simulink model "test_increase_button_laterelease"  (R2022b)
settings: Solver=FixedStepAuto  StartTime=0.0  StopTime=240  FixedStep=0.1  RelTol=1e-3
settings Model: Creator=cristian  LastModifiedBy=cristian
settings ConfigComp: CovEnable=on  RecordCoverage=on  CovModelRefEnable=on

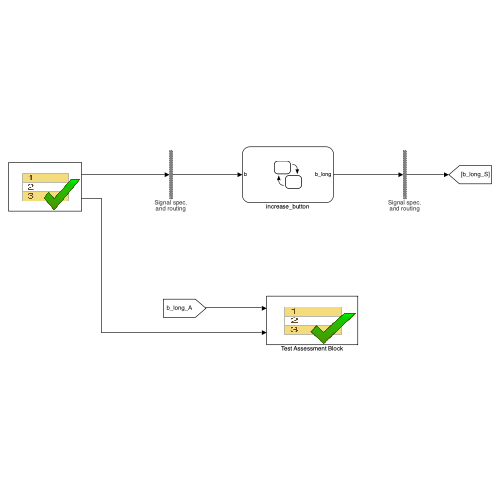
[thumbnail: Simulink's stored preview of the top-level diagram]
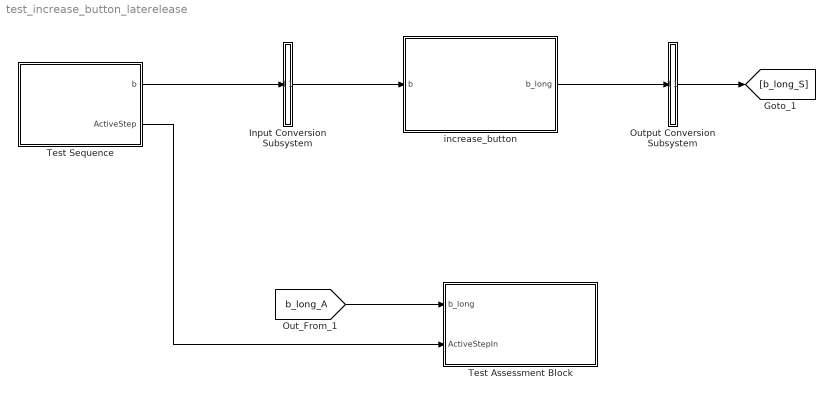
== system test_increase_button_laterelease ==
  Input Conversion Subsystem : Subsystem  Tag=__SLT_ICS__  Description=|
      | Signal spec.
      | and routing
      settings: AttributesFormatString=%<Description>
  Output Conversion Subsystem : Subsystem  Tag=__SLT_OCS__  Description=|
      | Signal spec.
      | and routing
      settings: AttributesFormatString=%<Description>
  Test Assessment Block : Test Sequence  Tag=__SLT_ASMT__  TreatAsAtomicUnit=on
  Test Sequence : Test Sequence  TreatAsAtomicUnit=on
  increase_button : Stateflow chart  TreatAsAtomicUnit=on
  wires:
  Test Sequence/1(b) -> Input Conversion Subsystem/1(Inport_1)
  Output Conversion Subsystem/1(Outport_1) -> [b_long_S]
  Input Conversion Subsystem/1(Outport_1) -> increase_button/1(b)
  increase_button/1(b_long) -> Output Conversion Subsystem/1(Inport_1)
  Test Sequence/2(ActiveStep) -> Test Assessment Block/2(ActiveStepIn)
  [b_long_A] -> Test Assessment Block/1(b_long)

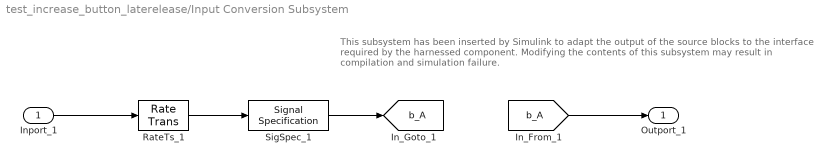
== system test_increase_button_laterelease/Input Conversion Subsystem ==
  note: This subsystem has been inserted by Simulink to adapt the output of the source blocks to the interface required by the harnessed component.
      |  Modifying the contents of this subsystem may result in compilation and simulation failure.
  Inport_1 : Inport
  RateTs_1 : RateTransition  OutPortSampleTime=[-1, 0]
  SigSpec_1 : SignalSpecification  OutDataTypeStr=boolean  Dimensions=[1]  SampleTime=[-1, 0]
  Outport_1 : Outport
  tag scope: b_A=global
  wires:
  [b_A] -> Outport_1/1
  SigSpec_1/1 -> [b_A]
  RateTs_1/1 -> SigSpec_1/1
  Inport_1/1 -> RateTs_1/1

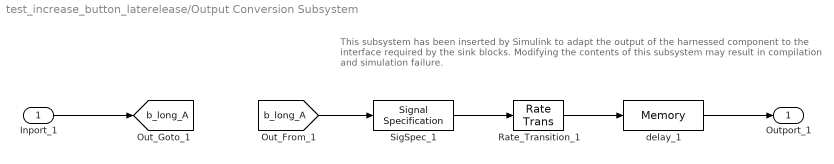
== system test_increase_button_laterelease/Output Conversion Subsystem ==
  note: This subsystem has been inserted by Simulink to adapt the output of the harnessed component to the interface required by the sink blocks.
      |  Modifying the contents of this subsystem may result in compilation and simulation failure.
  Inport_1 : Inport
  Rate_Transition_1 : RateTransition  OutPortSampleTimeOpt=Inherit
  SigSpec_1 : SignalSpecification  OutDataTypeStr=boolean  Dimensions=[1]
  delay_1 : Memory
  Outport_1 : Outport
  tag scope: b_long_A=global
  wires:
  Inport_1/1 -> [b_long_A]
  [b_long_A] -> SigSpec_1/1
  SigSpec_1/1 -> Rate_Transition_1/1
  Rate_Transition_1/1 -> delay_1/1
  delay_1/1 -> Outport_1/1

== stateflow chart test_increase_button_laterelease/Test Assessment Block ==
  state LateRelease
    state Run
      settings: description=Esecuzione test
      state Verify_LR_Init
        verify(b_long == 1);
        settings: description=Inizialmente il pulsante non è premuto.
      state Verify_LR_ButtonPressed
        settings: description=Viene premuto il pulsante.
        state Verify_LR_ButtonPressed_1
          verify(b_long == 1);
          settings: description=Fino a che non passa 1 secondo, non viene rilevato alcun cambiamento nella potenza.
        state Verify_LR_ButtonPressed_2
          verify(b_long == 0);
          settings: description=Viene rilevata la pressione lunga.
        state Verify_LR_ButtonPressed_3
          verify(b_long == 1);
          settings: description=La pressione lunga viene resettata.
        (default) -> Verify_LR_ButtonPressed_1
        Verify_LR_ButtonPressed_1 -> Verify_LR_ButtonPressed_2 : [
            | after(1,sec)
            | ]
        Verify_LR_ButtonPressed_2 -> Verify_LR_ButtonPressed_3 : [
            | after(sampleTime,sec)
            | ]
      state Verify_LR_ButtonReleased
        verify(b_long == 1);
        settings: description=Quando il pulsante viene rilasciato la pressione lunga non è verificata.
      state step_1_2
      (junction 471) -> (junction 474) [order 2]
      (junction 462) -> (junction 470) [order 2]
      Run -> (junction 445)
      (default) -> (junction 445)
      (junction 445) -> (junction 446) [order 1] : [ActiveStepIn == ActiveStepEnumH1.LR_Init
          | ]
      (junction 446) -> Verify_LR_Init [order 1] : [~in(LateRelease.Run.Verify_LR_Init)]
      (junction 445) -> (junction 454) [order 2]
      (junction 446) -> (junction 449) [order 2]
      (junction 454) -> (junction 455) [order 1] : [ActiveStepIn == ActiveStepEnumH1.LR_ButtonPressed
          | ]
      (junction 455) -> Verify_LR_ButtonPressed [order 1] : [~in(LateRelease.Run.Verify_LR_ButtonPressed)]
      (junction 454) -> (junction 462) [order 2]
      (junction 455) -> (junction 458) [order 2]
      (junction 462) -> (junction 463) [order 1] : [ActiveStepIn == ActiveStepEnumH1.LR_ButtonReleased
          | ]
      (junction 463) -> Verify_LR_ButtonReleased [order 1] : [~in(LateRelease.Run.Verify_LR_ButtonReleased)]
      (junction 463) -> (junction 466) [order 2]
      (junction 470) -> (junction 471)
      (junction 471) -> step_1_2 [order 1] : [~in(LateRelease.Run.step_1_2)]
    (default) -> Run
  (default) -> LateRelease : {assert(Active_Scenario_Index == 1,'The value of Scenario Parameter ''Active_Scenario_Index'' is not valid. Use the index of the scenario to specify it.')}
  data: b_long input boolean size=[1]; ActiveStepIn input; Active_Scenario_Index parameter =1; sampleTime constant double =str2num(get_param('InductionCooker','FixedStep'))

== stateflow chart test_increase_button_laterelease/Test Sequence ==
  settings: updateMethod=DISCRETE  sampleTime=0.1
  state LateRelease
    state LR_Init
      %% Initialize data outputs.
      b = true;
      settings: description=|
          | Pulsante non premuto.
          | Il pulsante lavora in logica negata come avviene per il bottone presente sulla scheda.
    state LR_ButtonPressed
      b = false
      settings: description=|
          | Pulsante premuto.
          | Lo stato passa da Wait a Pressed e da Pressed a LongPressed.
          | Consideriamo questo step attivo per più di 1 secondo (ad esempio un secondo e mezzo).
    state LR_ButtonReleased
      b = true
      settings: description=|
          | Pulsante rilasciato dopo un secondo e mezzo.
          | Lo stato passa da LongPressed a Wait.
    (default) -> LR_Init
    LR_Init -> LR_ButtonPressed : [
        | true
        | ]
    LR_ButtonPressed -> LR_ButtonReleased : [
        | after(1.5,sec)
        | ]
  (default) -> LateRelease : {assert(Active_Scenario_Index == 1,'The value of Scenario Parameter ''Active_Scenario_Index'' is not valid. Use the index of the scenario to specify it.')}
  data: b output boolean size=[1]; ActiveStep output Enum: ActiveStepEnumH1; sampleTime constant double =str2num(get_param('InductionCooker','FixedStep')); Active_Scenario_Index parameter =1

== stateflow chart test_increase_button_laterelease/increase_button ==
  note: Bottone a livelli, la pressione per un numero di secondi pari a DURATION permette di avere un uscita alta in maniera istantanea.
      | Per avere in output un valore PRESSED, è necessare lasciare il bottone e premere tra un output e l'altro.
  state Wait
    en: b_long = RELEASED
  state Pressed
    en: b_long = RELEASED;
    on after(DURATION,sec): b_long = PRESSED
  state LongPressed
    en: b_long = RELEASED
  (default) -> Wait
  Wait -> Pressed : [b == PRESSED]
  Pressed -> Wait [order 1] : [b == RELEASED]
  LongPressed -> Wait : [b == RELEASED]
  Pressed -> LongPressed [order 2] : [b_long == PRESSED && b == PRESSED]
  data: b_long output boolean size=1; PRESSED constant boolean size=1 =0; RELEASED constant boolean size=1 =1; b input boolean size=1; DURATION constant double size=1 =1
